simulink model "lab5_ASP_HudinaA_cop"  (R2022a)
settings: Solver=VariableStepAuto  StartTime=0.0  StopTime=1.0  RelTol=1e-3
libraries: dspsnks4 x1, dspvision x1, dspfdesign x1, dspsrcs4 x1, matrix_library x1
settings Model: Creator=Student  LastModifiedBy=Анастасия
settings SolverCC: AlgebraicLoopSolver=TrustRegion
settings DataIOCC: ReturnWorkspaceOutputs=off
settings DebuggingCC: UnconnectedInputMsg=warning  UnconnectedOutputMsg=warning  UnconnectedLineMsg=warning  SFMachineParentedDataDiag=warning  ArithmeticOperatorsInVariantConditions=warning
settings SFSimCC: CustomCodeUndefinedFunction=UseInterfaceOnly

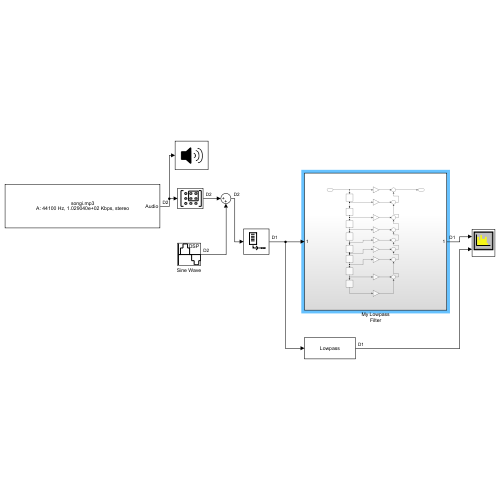
[thumbnail: Simulink's stored preview of the top-level diagram]
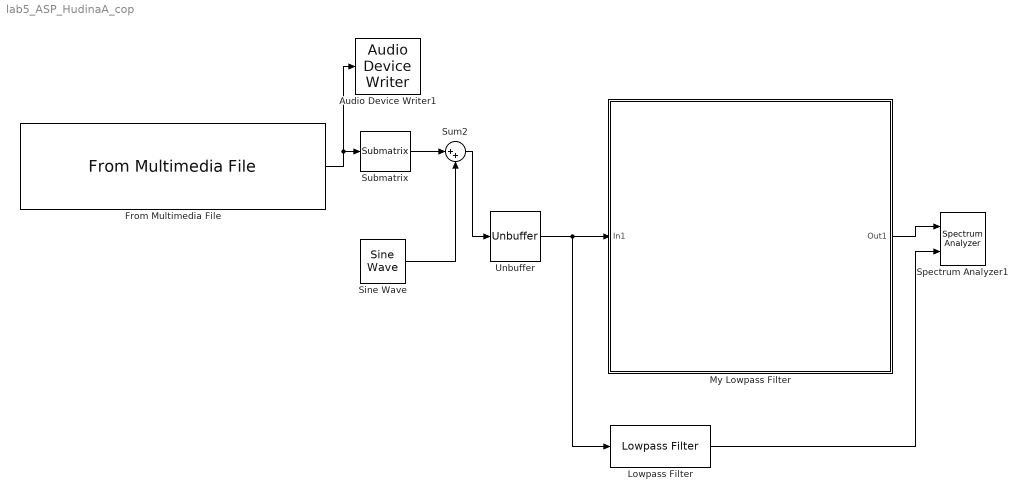
== system lab5_ASP_HudinaA_cop ==
  Audio Device Writer1 : dspsnks4/Audio Device Writer  Driver=DirectSound  Device=Default  InheritSampleRate=on  SampleRate=44100  BitDepth=16-bit integer  BufferSize=4096  NumBuffers=10  DefaultOutputChannelMapping=on  OutputChannelMapping=1:2  OutputNumUnderrunSamples=off  DriverIdx=1  DeviceWarnFlag=''
  From Multimedia File : dspvision/From Multimedia File  inputFilename=C:\Users\Анастасия\Documents\MATLAB\MATLAB_labs\lab1\songi.mp3  readRange=[1 Inf]  loop=on  numPlays=inf  outputStreams=Audio only  videoDataType=single  audioDataType=double  inheritSampleTime=on  userDefinedSampleTime=1/30  noAudioOutput=off  isIntensityVideo=off  fourcc=RGB  colorVideoFormat=Separate color signals  outputEOF=off  dataOrg=Column-major  audioFrameSize=1024  computeAudioFrameSize=off  outSamplingMode=Sample based
  Lowpass Filter : dspfdesign/Lowpass Filter  FilterType=FIR  DesignForMinimumOrder=off  FilterOrder=8  PassbandFrequency=14e3  StopbandFrequency=12e3  PassbandRipple=0.1  StopbandAttenuation=80  InheritSampleRate=off  SampleRate=44100  SimulateUsing=Interpreted execution  roundingMode=Floor  coeffsDataTypeStr=fixdt(1,16)
  My Lowpass Filter : Subsystem
  Sine Wave : dspsrcs4/Sine Wave  Amplitude=0  Frequency=17000  Phase=0  SampleMode=Discrete  OutComplex=Real  CompMethod=Trigonometric fcn  TableSize=Speed  SampleTime=1/44100  SamplesPerFrame=1024  ResetState=Restart at time zero  OutputFrames=off  dataType=double  wordLen=16  udDataType=sfix(16)  fracBitsMode=Best precision  numFracBits=15  OutDataTypeStr=double  LastOutDataTypeStr=double
  Spectrum Analyzer1 : SpectrumAnalyzer  NumInputPorts=2
  Submatrix : matrix_library/Submatrix  RowSpan=Range of rows  RowStartMode=First  RowStartIndex=1  RowEndMode=Last  RowEndIndex=1  ColSpan=One column  ColStartMode=First  ColStartIndex=1  ColEndMode=Last  ColEndIndex=1
      settings: SourceProductBaseCode=SL
  Sum2 : Sum  Inputs=|++
  Unbuffer : Unbuffer
  wires:
  Unbuffer/1 -> My Lowpass Filter/1(In1), Lowpass Filter/1
  Lowpass Filter/1 -> Spectrum Analyzer1/2
  My Lowpass Filter/1(Out1) -> Spectrum Analyzer1/1
  From Multimedia File/1 -> Audio Device Writer1/1, Submatrix/1
  Sine Wave/1 -> Sum2/2
  Submatrix/1 -> Sum2/1
  Sum2/1 -> Unbuffer/1

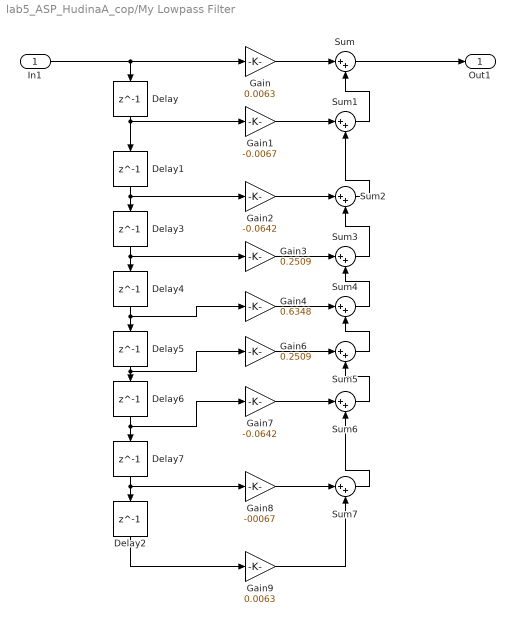
== system lab5_ASP_HudinaA_cop/My Lowpass Filter ==
  In1 : Inport
  Delay{,1..7} (8 alike) : Delay  DelayLength=1  InitialCondition=0
  Gain : Gain  Gain=0.0063
  Gain1 : Gain  Gain=-0.0067
  Gain2 : Gain  Gain=-0.0642
  Gain3 : Gain  Gain=0.2509
  Gain4 : Gain  Gain=0.6348
  Gain6 : Gain  Gain=0.2509
  Gain7 : Gain  Gain=-0.0642
  Gain8 : Gain  Gain=-00067
  Gain9 : Gain  Gain=0.0063
  Sum{,1..7} (8 alike) : Sum  Inputs=|++
  Out1 : Outport  VectorParamsAs1DForOutWhenUnconnected=off
  wires:
  Sum6/1 -> Sum5/2
  Delay7/1 -> Gain8/1, Delay2/1
  Delay3/1 -> Gain3/1, Delay4/1
  Sum/1 -> Out1/1
  Sum7/1 -> Sum6/2
  Gain3/1 -> Sum3/1
  Delay/1 -> Delay1/1, Gain1/1
  Gain8/1 -> Sum7/1
  Delay5/1 -> Gain6/1, Delay6/1
  Delay4/1 -> Gain4/1, Delay5/1
  Gain/1 -> Sum/1
  Sum1/1 -> Sum/2
  Delay6/1 -> Gain7/1, Delay7/1
  Delay2/1 -> Gain9/1
  Gain9/1 -> Sum7/2
  Delay1/1 -> Gain2/1, Delay3/1
  Gain1/1 -> Sum1/1
  Gain6/1 -> Sum5/1
  Sum3/1 -> Sum2/2
  Gain2/1 -> Sum2/1
  Sum2/1 -> Sum1/2
  Gain7/1 -> Sum6/1
  Sum4/1 -> Sum3/2
  Gain4/1 -> Sum4/1
  Sum5/1 -> Sum4/2
  In1/1 -> Delay/1, Gain/1
